simulink model "Rocky"  (R2021a)
settings: Solver=VariableStepAuto  StartTime=0.0  StopTime=10.0  RelTol=1e-3
values from neighbouring files (symbols this model uses):
  a = 1/17.48    (= 0.0572082379863)    [Rocky_5_closed_loop_poles.m]
  b = 0.0031    [Rocky_5_closed_loop_poles.m]
  Ci = double(solutions.Ci)    [Rocky_5_closed_loop_poles.m]
  g = 9.81    [Rocky_5_closed_loop_poles.m]
  Ji = double(solutions.Ji)    [Rocky_5_closed_loop_poles.m]
  Jp = double(solutions.Jp)    [Rocky_5_closed_loop_poles.m]
  Ki = double(solutions.Ki)    [Rocky_5_closed_loop_poles.m]
  Kp = double(solutions.Kp)    [Rocky_5_closed_loop_poles.m]
  l = 0.362    [Rocky_5_closed_loop_poles.m]
settings Model: Creator=jliu2  LastModifiedBy=jliu2

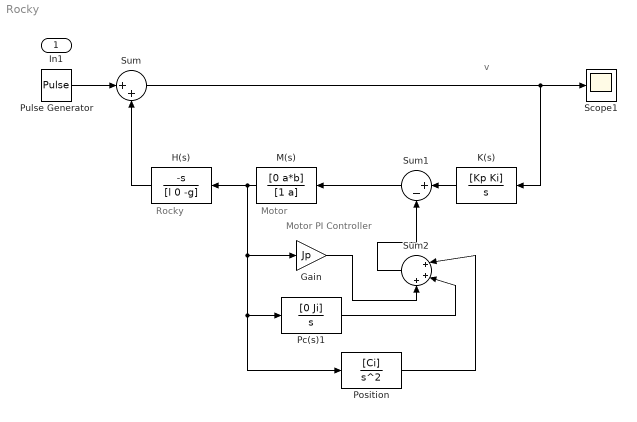
== system Rocky ==
  note: v
  note: Motor
  note: Rocky
  note: Motor PI Controller
  In1 : Inport
  Gain : Gain  Gain=Jp
  H(s) : TransferFcn  Numerator=[-1 0]  Denominator=[l 0 -g]
  K(s) : TransferFcn  Numerator=[Kp Ki]  Denominator=[1 0]
  M(s) : TransferFcn  Numerator=[0 a*b]  Denominator=[1 a]
  Pc(s)1 : TransferFcn  Numerator=[0 Ji]  Denominator=[1 0]
  Position : TransferFcn  Numerator=[Ci]  Denominator=[1 0 0]
  Pulse Generator : DiscretePulseGenerator  PulseType=Time based  Period=10  PulseWidth=0.1  PhaseDelay=.5
  Scope1 : Scope
  Sum : Sum  Inputs=|++
  Sum1 : Sum  Inputs=|+-
  Sum2 : Sum  Inputs=|+++
  wires:
  Pulse Generator/1 -> Sum/1
  Sum/1 -> K(s)/1, Scope1/1
  M(s)/1 -> Position/1, Pc(s)1/1, Gain/1, H(s)/1
  H(s)/1 -> Sum/2
  K(s)/1 -> Sum1/1
  Sum1/1 -> M(s)/1
  Position/1 -> Sum2/1
  Gain/1 -> Sum2/3
  Pc(s)1/1 -> Sum2/2
  Sum2/1 -> Sum1/2
